simulink model "sepicmm_vs_sepicsm"  (R2015a)
settings: Solver=ode45  StartTime=0.0  StopTime=1  RelTol=1e-3
values from neighbouring files (symbols this model uses):
  alpha = min(d1,d2)    [Final_2.m]    (also in Final_discreto.m)
  Ao = Aaum-L*Caum    [Final_2.m]
  Bo = [Baum L]    [Final_2.m]
  C1 = 190e-6    (= 0.00019)    [Final_2.m]    (also in Final_discreto.m = 0.0022)
  C2 = 190e-6    (= 0.00019)    [Final_2.m]    (also in Final_discreto.m = 0.0022)
  Co = [eye(size(Ao,1)-1) zeros(size(Ao,1)-1,1)]    [Final_2.m]
  Do = zeros(size(Ao,1)-1,2)    [Final_2.m]
  E0 = 20    [Final_2.m]    (also in Final_discreto.m = 36)
  ki = Ki_(5,1)    [Final_2.m]
  ks = [Ki_(1,1) Ki_(2,1) Ki_(3,1) Ki_(4,1) ]'    [Final_2.m]
  L1 = 2.3e-3    (= 0.0023)    [Final_2.m]    (also in Final_discreto.m = 0.00156)
  L2 = 330e-6    (= 0.00033)    [Final_2.m]    (also in Final_discreto.m = 0.00324)
  R0 = 44    [Final_2.m]    (also in Final_discreto.m = 50)
  R1 = 2.134    [Final_2.m]    (also in Final_discreto.m = 0.3)
  R2 = 0.234    [Final_2.m]    (also in Final_discreto.m = 0.3)
  V0 = 20    [Final_2.m]    (also in Final_discreto.m = 120)
libraries: powerlib x11, powerlib_meascontrol x1
settings Model: Creator=berme_000  LastModifiedBy=berme_000

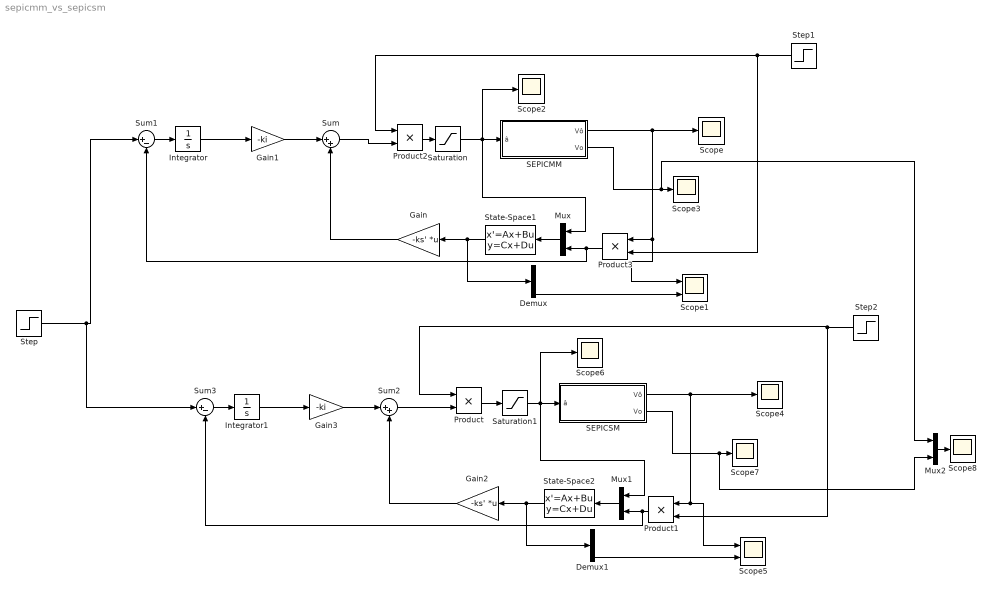
== system sepicmm_vs_sepicsm ==
  Demux : Demux
  Demux1 : Demux
  Gain : Gain  Gain=-ks'  Multiplication=Matrix(K*u)
  Gain1 : Gain  Gain=-ki
  Gain2 : Gain  Gain=-ks'  Multiplication=Matrix(K*u)
  Gain3 : Gain  Gain=-ki
  Integrator : Integrator
  Integrator1 : Integrator
  Mux : Mux  Inputs=2
  Mux1 : Mux  Inputs=2
  Mux2 : Mux  Inputs=2
  Product{,1..3} (4 alike) : Product
  "SEPICMM " : Subsystem
  "SEPICSM " : Subsystem
  Saturation : Saturate  UpperLimit=1-alpha  LowerLimit=0.5-alpha
  Saturation1 : Saturate  UpperLimit=1-alpha  LowerLimit=0.5-alpha
  Scope{,2..4,6..8} (7 alike) : Scope
      Scope settings: YMin=-4.25e-09  YMax=-2.5e-10
      Scope2 settings: YMin=0.216701  YMax=0.216701  SaveName=ScopeData3
      Scope3 settings: TimeRange=1  YMin=75  YMax=140  SaveName=ScopeData4
      Scope4 settings: YMin=-2.5  YMax=42.5  SaveName=ScopeData5
      Scope6 settings: YMin=-1  YMax=1  SaveName=ScopeData7
      Scope7 settings: TimeRange=1  YMin=52.525  YMax=52.95  SaveName=ScopeData8
      Scope8 settings: YMin=0  YMax=170  SaveName=ScopeData9
  Scope1 : Scope  NumInputPorts=2
      settings: YMin=-120~-119.98  YMax=-120~-119.86
  Scope5 : Scope  NumInputPorts=2
      settings: YMin=-120~-119.98  YMax=-120~-119.86  SaveName=ScopeData6
  State-Space1 : StateSpace  A=Ao  B=Bo  C=Co  D=Do  X0=0
  State-Space2 : StateSpace  A=Ao  B=Bo  C=Co  D=Do  X0=0
  Step : Step  Time=0.5  After=40  SampleTime=0
  Step1 : Step  Time=0.08  SampleTime=0
  Step2 : Step  Time=0.08  SampleTime=0
  Sum : Sum  Inputs=|++
  Sum1 : Sum  Inputs=|+-
  Sum2 : Sum  Inputs=|++
  Sum3 : Sum  Inputs=|+-
  wires:
  Mux/1 -> State-Space1/1
  State-Space1/1 -> Demux/1, Gain/1
  Integrator/1 -> Gain1/1
  Gain1/1 -> Sum/1
  Gain/1 -> Sum/2
  Demux/4 -> Scope1/2
  "SEPICMM "/2(Vo) -> Mux2/1, Scope3/1
  Saturation/1 -> Scope2/1, "SEPICMM "/1(â), Mux/1
  "SEPICMM "/1(Vô) -> Scope1/1, Product3/1, Scope/1
  Sum1/1 -> Integrator/1
  "SEPICSM "/1(Vô) -> Product1/1, Scope5/1, Scope4/1
  Mux1/1 -> State-Space2/1
  Sum2/1 -> Product/2
  State-Space2/1 -> Demux1/1, Gain2/1
  Integrator1/1 -> Gain3/1
  Gain3/1 -> Sum2/1
  Gain2/1 -> Sum2/2
  Demux1/4 -> Scope5/2
  Step2/1 -> Product1/2, Product/1
  "SEPICSM "/2(Vo) -> Mux2/2, Scope7/1
  Saturation1/1 -> Scope6/1, Mux1/1, "SEPICSM "/1(â)
  Product1/1 -> Sum3/2, Mux1/2
  Step/1 -> Sum3/1, Sum1/1
  Sum3/1 -> Integrator1/1
  Product/1 -> Saturation1/1
  Mux2/1 -> Scope8/1
  Product3/1 -> Sum1/2, Mux/2
  Step1/1 -> Product3/2, Product2/1
  Product2/1 -> Saturation/1
  Sum/1 -> Product2/2

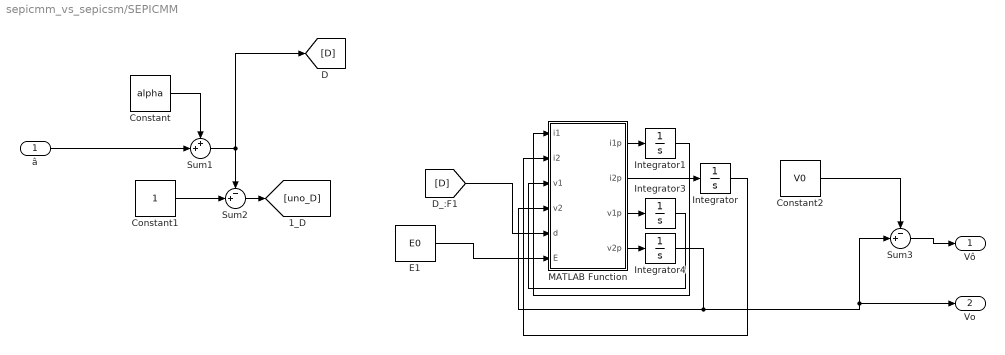
== system sepicmm_vs_sepicsm/SEPICMM  ==
  â : Inport
  Constant : Constant  Value=alpha
  Constant1 : Constant
  Constant2 : Constant  Value=V0
  E1 : Constant  Value=E0
  Integrator{,1,3..4} (4 alike) : Integrator
  MATLAB Function : MATLAB Function  TreatAsAtomicUnit=on
  Sum1 : Sum  Inputs=++|
  Sum2 : Sum  Inputs=-+|
  Sum3 : Sum  Inputs=-+|
  Vô : Outport
  Vo : Outport  Port=2
  wires:
  Sum1/1 -> [D], Sum2/1
  Constant/1 -> Sum1/1
  Constant1/1 -> Sum2/2
  Constant2/1 -> Sum3/1
  Sum3/1 -> Vô/1
  Sum2/1 -> [uno_D]
  â/1 -> Sum1/2
  E1/1 -> MATLAB Function/6(E)
  [D] -> MATLAB Function/5(d)
  MATLAB Function/2(i2p) -> Integrator/1
  MATLAB Function/1(i1p) -> Integrator1/1
  MATLAB Function/4(v2p) -> Integrator4/1
  MATLAB Function/3(v1p) -> Integrator3/1
  Integrator1/1 -> MATLAB Function/1(i1)
  Integrator/1 -> MATLAB Function/2(i2)
  Integrator3/1 -> MATLAB Function/3(v1)
  Integrator4/1 -> Vo/1, Sum3/2, MATLAB Function/4(v2)

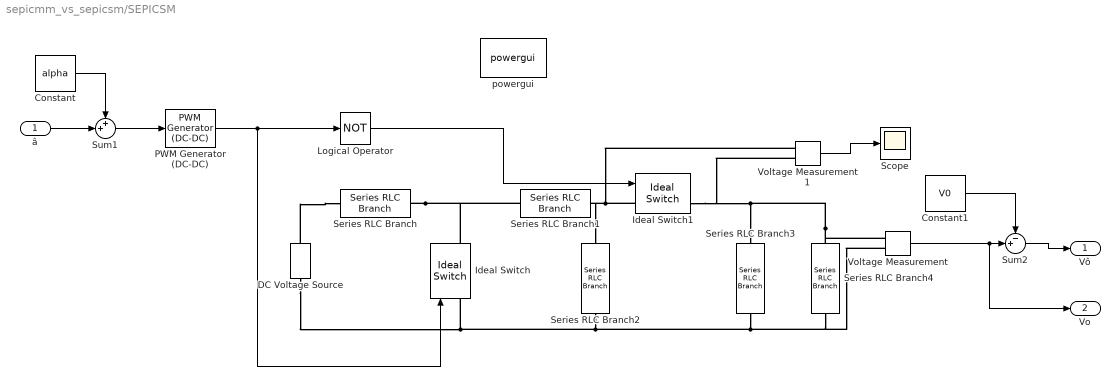
== system sepicmm_vs_sepicsm/SEPICSM  ==
  â : Inport
  Constant : Constant  Value=alpha
  Constant1 : Constant  Value=V0
  DC Voltage Source : powerlib/Electrical Sources/DC Voltage Source  Amplitude=E0  Measurements=None
  Ideal Switch : powerlib/Power Electronics/Ideal Switch  Ron=0.001  Lon=0  IC=0  Rs=1e5  Cs=inf  Measurements=on
  Ideal Switch1 : powerlib/Power Electronics/Ideal Switch  Ron=0.001  Lon=0  IC=0  Rs=1e5  Cs=inf  Measurements=on
  Logical Operator : Logic  Operator=NOT  AllPortsSameDT=off  OutDataTypeStr=boolean
  PWM Generator (DC-DC) : powerlib_meascontrol/Pulse & Signal Generators/PWM Generator (DC-DC)  Fsw=50000  Ts=0
  Scope : Scope
      settings: YMin=-9.23568e-13  YMax=-9.23568e-13  SaveName=ScopeData2
  Series RLC Branch : powerlib/Elements/Series RLC Branch  LConnTagsString=__new0  RConnTagsString=__new0  BranchType=RL  Resistance=R1  Inductance=L1  SetiL0=on  InitialCurrent=0  Capacitance=1e-6  Setx0=off  InitialVoltage=0  Measurements=None
  Series RLC Branch1 : powerlib/Elements/Series RLC Branch  LConnTagsString=__new0  RConnTagsString=__new0  BranchType=C  Resistance=1  Inductance=L1  SetiL0=off  InitialCurrent=0  Capacitance=C1  Setx0=on  InitialVoltage=0  Measurements=None
  Series RLC Branch2 : powerlib/Elements/Series RLC Branch  LConnTagsString=__new0  RConnTagsString=__new0  BranchType=RL  Resistance=R2  Inductance=L2  SetiL0=on  InitialCurrent=0  Capacitance=1e-6  Setx0=off  InitialVoltage=0  Measurements=None
  Series RLC Branch3 : powerlib/Elements/Series RLC Branch  LConnTagsString=__new0  RConnTagsString=__new0  BranchType=C  Resistance=1  Inductance=L1  SetiL0=off  InitialCurrent=0  Capacitance=C2  Setx0=on  InitialVoltage=0  Measurements=None
  Series RLC Branch4 : powerlib/Elements/Series RLC Branch  LConnTagsString=__new0  RConnTagsString=__new0  BranchType=R  Resistance=R0  Inductance=L1  SetiL0=off  InitialCurrent=0  Capacitance=1e-6  Setx0=off  InitialVoltage=0  Measurements=None
  Sum1 : Sum  Inputs=++|
  Sum2 : Sum  Inputs=-+|
  Voltage Measurement : powerlib/Measurements/Voltage Measurement  PhasorSimulation=off  OutputType=Complex  PSBequivalent=0
  Voltage Measurement1 : powerlib/Measurements/Voltage Measurement  PhasorSimulation=off  OutputType=Complex  PSBequivalent=0
  powergui : powerlib/powergui  Priority=1  SimulationMode=Continuous  SolverType=Tustin  SampleTime=50e-6  frequency=60  SPID=off  DisableSnubberDevices=off  DisableRonSwitches=off  DisableVfSwitches=off  SwTol=0  DisplayEquations=off  Interpol=off  methode=off  Ts=0  FunctionMessages=off  echomessages=off  HookPort=off  EnableUseOfTLC=off  x0status=blocks  frequencyindice=0  Pbase=100e6  ErrMax=1e-4  Iterations=50  UnitsV=kV  UnitsW=MW  buscounter=0  RestoreLinks=warning  ResistiveCurrentMeasurement=off  Frange=[0:2:500]  Ylog=off  Xlog=on  ShowGrid=off  save=off  variable=ZData  structure=0  ZoomFFT=off  StartTime=0.0  cycles=1  DisplayStyle=1  fundamental=60  FreqAxis=off  MaxFrequency=1000  frequencyindicesteady=1  RmsSteady=1  display=off
  Vô : Outport
  Vo : Outport  Port=2
  wires:
  â/1 -> Sum1/2
  Sum1/1 -> PWM Generator (DC-DC)/1
  Constant/1 -> Sum1/1
  PWM Generator (DC-DC)/1 -> Logical Operator/1, Ideal Switch/1
  Logical Operator/1 -> Ideal Switch1/1
  Voltage Measurement1/1 -> Scope/1
  Constant1/1 -> Sum2/1
  Voltage Measurement/1 -> Vo/1, Sum2/2
  Sum2/1 -> Vô/1
  connections:
  Series RLC Branch/RConn1 -- Series RLC Branch1/LConn1 -- Ideal Switch/RConn1
  Ideal Switch1/LConn1 -- Series RLC Branch1/RConn1 -- Series RLC Branch2/RConn1 -- Voltage Measurement1/LConn1
  Series RLC Branch2/LConn1 -- DC Voltage Source/LConn1 -- Ideal Switch/LConn1 -- Series RLC Branch3/RConn1 -- Voltage Measurement/LConn2 -- Series RLC Branch4/RConn1
  Voltage Measurement/LConn1 -- Series RLC Branch4/LConn1 -- Series RLC Branch3/LConn1 -- Ideal Switch1/RConn1 -- Voltage Measurement1/LConn2
  DC Voltage Source/RConn1 -- Series RLC Branch/LConn1

== matlab function sepicmm_vs_sepicsm/SEPICMM /MATLAB Function ==
  data: i1 input; i2 input; v1 input; v2 input; i1p output; d input; E input; i2p output; v1p output; v2p output
function [i1p,i2p,v1p,v2p]  = fcn(i1,i2,v1,v2,d,E)
%#codegen
l1=1.56e-3;
l2=3.24e-3;
r0=50;
r1=0.3;
r2=0.3;
c1=2.2e-3;
c2=2.2e-3;
i1p=(E-i1*r1-(1-d)*(v1+v2))/l1;
i2p=(-v1*d+(1-d)*v2-i2*r2)/l2;
v1p=(i2*d+i1*(1-d))/c1;
v2p=(-v2/r0+(1-d)*(i1-i2))/c2;
